simulink model "LF_Controller"  (R2024a)
settings: configuration reference "csMultiInstance" (kept outside this file)
Description:
  | Lane following controller (SW component)
settings Model: DataDictionary=DD_LF_Controller.sldd  EnableAccessToBaseWorkspace=off  Creator=The MathWorks, Inc.  LastModifiedBy=The MathWorks, Inc.
settings ConfigSetRef: SourceName=csMultiInstance

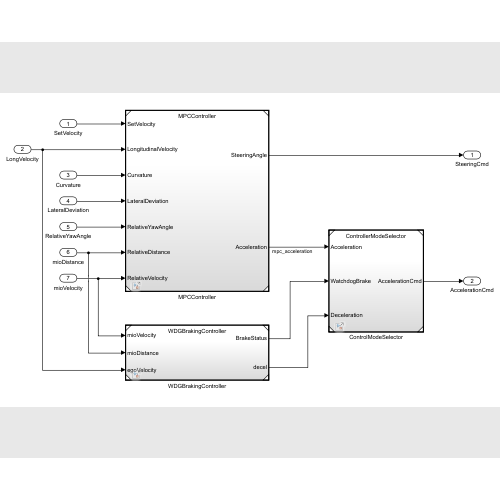
[thumbnail: Simulink's stored preview of the top-level diagram]
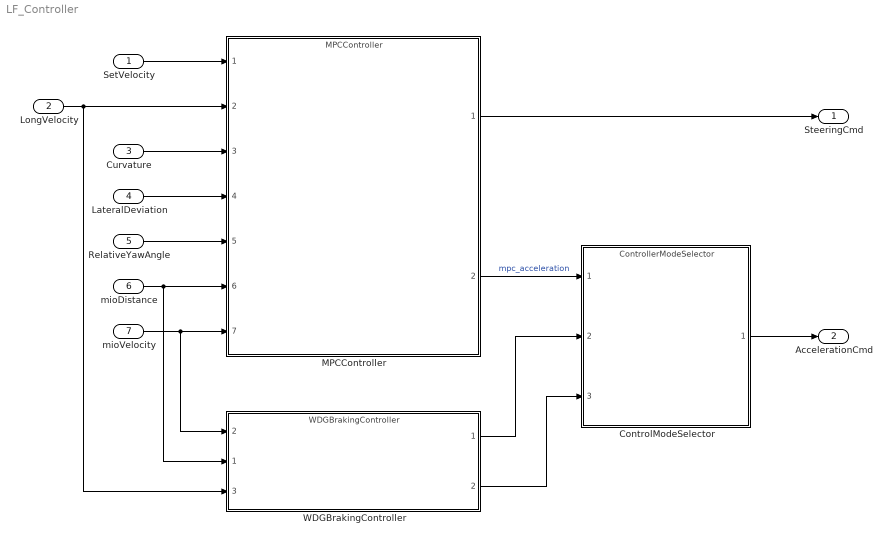
== system LF_Controller ==
  SetVelocity : Inport
  LongVelocity : Inport  Port=2
  Curvature : Inport  Port=3
  LateralDeviation : Inport  Port=4
  RelativeYawAngle : Inport  Port=5
  mioDistance : Inport  Port=6
  mioVelocity : Inport  Port=7
  ControlModeSelector : ModelReference  ModelNameDialog=ControllerModeSelector  SimulationMode=Normal  ModelReferenceVersion=8.0
  MPCController : ModelReference  ModelNameDialog=MPCController  SimulationMode=Normal  ModelReferenceVersion=8.0
  WDGBrakingController : ModelReference  ModelNameDialog=WDGBrakingController  SimulationMode=Normal  ModelReferenceVersion=8.0
      settings: PortSchema="{\"entries\":[{\"content\":{\"sides\":[{\"content\":{\"connectorIds\":[\"In2\",\"In1\",\"In3\"]},\"type\":\"ConnectorPlacement.EquallySpacedRectSide\",\"uuid\":\"57705aa4-366f-4978-8b4b-15f74a9aab94\"},{\"content\":{\"connectorIds\":[\"Out1\",\"Out2\"],\"side\":\"RIGHT\"},\"type\":\"ConnectorPlacement.EquallySpacedRectSide\",\"uuid\":\"9c18fe49-6c00-4be7-8985-e5ee85291c64\"},{\"content\":{\"connectorIds\":[],\"side\":\"TOP\"},\"type\":\"ConnectorPlacement.EquallySpacedRectSide\",\"uuid\":\"ebf1e965-1620-4f1d-9314-76deb949cadd\"},{\"content\":{\"connectorIds\":[],\"side\":\"HIDDEN\"},\"type\":\"ConnectorPlacement.EquallySpacedRectSide\",\"uuid\":\"c9194109-8624-4ca2-94ec-703cbf1a4433\"}]},\"type\":\"ConnectorPlacement.EquallySpacedConnector\",\"uuid\":\"c9b9c9f8-434c-4c2b-a6c6-10427f2ee2b9\"}],\"packageUris\":[\"http://schema.mathworks.com/mf0/Connector/R2020b\"],\"version\":\"1.0\"}"
  SteeringCmd : Outport
  AccelerationCmd : Outport  Port=2
  wires:
  mioDistance/1 -> WDGBrakingController/1, MPCController/6
  SetVelocity/1 -> MPCController/1
  Curvature/1 -> MPCController/3
  MPCController/1 -> SteeringCmd/1
  LateralDeviation/1 -> MPCController/4
  RelativeYawAngle/1 -> MPCController/5
  LongVelocity/1 -> WDGBrakingController/3, MPCController/2
  ControlModeSelector/1 -> AccelerationCmd/1
  MPCController/2 -> ControlModeSelector/1  "mpc_acceleration"
  mioVelocity/1 -> WDGBrakingController/2, MPCController/7
  WDGBrakingController/2 -> ControlModeSelector/3
  WDGBrakingController/1 -> ControlModeSelector/2
